simulink model "eg_6_05_R2020a"  (R2020a)
settings: Solver=ode4  StartTime=0.0  StopTime=1  FixedStep=0.001  RelTol=1e-3  EnableMultiTasking=on
values from neighbouring files (symbols this model uses):
  A = [ 0  1  0  0 ... (first row only)    [eg_6_02.m]    (also in eg_6_03.m = [ 0   1; eg_6_04_1a.m = [ 0   1; eg_6_04_1b.m = [ 0   1; eg_6_04_1c.m = [ 0   1)
  Av = [    0       1       0       0 ... (first row only)    [eg_6_05c.m]    (also in eg_6_05d.m)
  B = [  0 ... (first row only)    [eg_6_05a.m]    (also in eg_6_05b.m; eg_6_05c.m; eg_6_05d.m)
  Bv = [  0 ... (first row only)    [eg_6_05c.m]    (also in eg_6_05d.m)
  C = [ 0  0  1  0 ]    [eg_6_05a.m]    (also in eg_6_05b.m; eg_6_05c.m; eg_6_05d.m)
  H = 10    [eg_6_05c.m]    (also in eg_6_05d.m)
  K = [ -7/2  -5/2  -13/2  -11/2 ]    [eg_6_05c.m]    (also in eg_6_05d.m)
  L = - Delta_A*inv(Vo)*e'    [eg_6_05a.m]    (also in eg_6_05b.m = Kd'; eg_6_05c.m = Kd'; eg_6_05d.m = Kd')
  x0 = [ 1 ... (first row only)    [eg_6_04_1c.m]    (also in eg_6_05c.m = [ -0.5; eg_6_05d.m = [ -0.5)
  x0_hat = [ 0 ... (first row only)    [eg_6_04_1c.m]    (also in eg_6_05c.m; eg_6_05d.m)
settings Model: Creator=kawata  LastModifiedBy=kawata
settings DataIOCC: LimitDataPoints=on  SaveFormat=Array  SignalLoggingSaveFormat=ModelDataLogs  ReturnWorkspaceOutputs=off
settings OptimizationCC: ExpressionDepthLimit=2147483647  LifeSpan=inf
settings DebuggingCC: UnderspecifiedInitializationDetection=Classic  MergeDetectMultiDrivingBlocksExec=none  SolverPrmCheckMsg=warning  FcnCallInpInsideContextMsg=warning  StateNameClashWarn=warning  SFUnexpectedBacktrackingDiag=warning  SFNoUnconditionalDefaultTransitionDiag=warning  SFExecutionAtInitializationDiag=none  ArithmeticOperatorsInVariantConditions=warning
settings HardwareCC: ProdBitPerPointer=32  ProdBitPerSizeT=32  ProdBitPerPtrDiffT=32  ProdLargestAtomicFloat=None  ProdIntDivRoundTo=Undefined  ProdEndianess=Unspecified  ProdWordSize=32  ProdHWDeviceType=32-bit Generic
settings ModelReferenceCC: PropagateSignalLabelsOutOfModel=off
settings SFSimCC: SimUseLocalCustomCode=off  CustomCodeUndefinedFunction=UseInterfaceOnly
settings RTWCC: RTWUseLocalCustomCode=off
settings CodeAppCC: StateflowObjectComments=on
settings GRTTargetCC: TargetLangStandard=C89/C90 (ANSI)  CombineOutputUpdateFcns=off  GRTInterface=on
settings ConfigComp: CovMetricSettings=dw  CovSaveCumulativeToWorkspaceVar=on  CovSaveSingleToWorkspaceVar=on  CovExternalEMLEnable=off

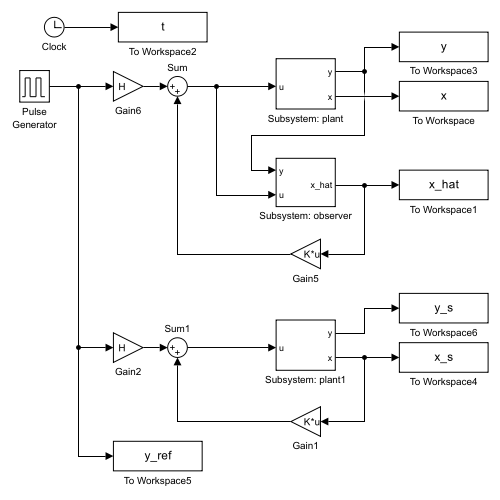
[thumbnail: Simulink's stored preview of the top-level diagram]
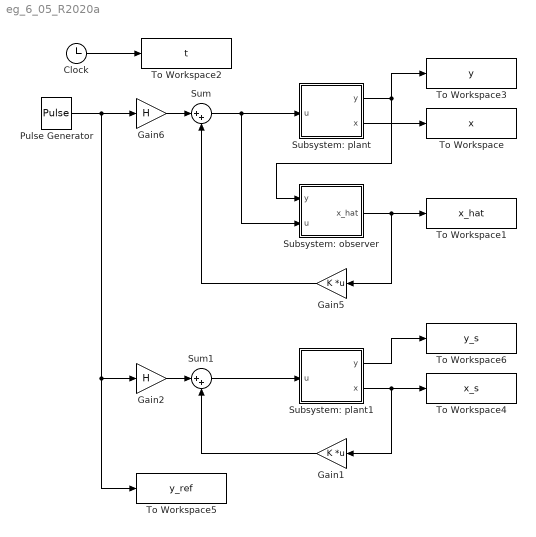
== system eg_6_05_R2020a ==
  Clock : Clock
  Gain1 : Gain  Gain=K  Multiplication=Matrix(K*u)
  Gain2 : Gain  Gain=H
  Gain5 : Gain  Gain=K  Multiplication=Matrix(K*u)
  Gain6 : Gain  Gain=H
  Pulse Generator : DiscretePulseGenerator  PulseType=Time based  Period=10  PulseWidth=50
  Subsystem: observer : Subsystem
  Subsystem: plant : Subsystem
  Subsystem: plant1 : Subsystem
  Sum : Sum  Inputs=|++  InputSameDT=on  SaturateOnIntegerOverflow=on  OutDataTypeStr=Inherit: Same as first input
  Sum1 : Sum  Inputs=|++  InputSameDT=on  SaturateOnIntegerOverflow=on  OutDataTypeStr=Inherit: Same as first input
  To Workspace : ToWorkspace  VariableName=x  SampleTime=-1
  To Workspace1 : ToWorkspace  VariableName=x_hat  SampleTime=-1
  To Workspace2 : ToWorkspace  VariableName=t  SampleTime=-1
  To Workspace3 : ToWorkspace  VariableName=y  SampleTime=-1
  To Workspace4 : ToWorkspace  VariableName=x_s  SampleTime=-1
  To Workspace5 : ToWorkspace  VariableName=y_ref  SampleTime=-1
  To Workspace6 : ToWorkspace  VariableName=y_s  SampleTime=-1
  wires:
  Clock/1 -> To Workspace2/1
  Sum/1 -> Subsystem: observer/2(u), Subsystem: plant/1(u)
  Subsystem: observer/1(x_hat) -> To Workspace1/1, Gain5/1
  Subsystem: plant/2(x) -> To Workspace/1
  Subsystem: plant/1(y) -> To Workspace3/1, Subsystem: observer/1(y)
  Pulse Generator/1 -> Gain6/1, To Workspace5/1, Gain2/1
  Gain6/1 -> Sum/1
  Gain5/1 -> Sum/2
  Sum1/1 -> Subsystem: plant1/1(u)
  Subsystem: plant1/2(x) -> To Workspace4/1, Gain1/1
  Subsystem: plant1/1(y) -> To Workspace6/1
  Gain2/1 -> Sum1/1
  Gain1/1 -> Sum1/2

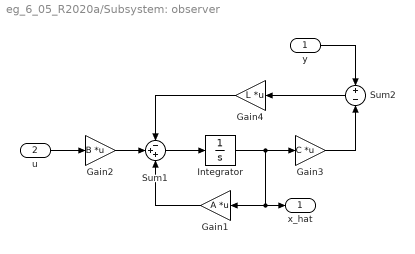
== system eg_6_05_R2020a/Subsystem: observer ==
  y : Inport
  u : Inport  Port=2
  Gain1 : Gain  Gain=A  Multiplication=Matrix(K*u)  SaturateOnIntegerOverflow=on  OutDataTypeStr=Inherit: Same as input  ParamDataTypeStr=Inherit: Same as input
  Gain2 : Gain  Gain=B  Multiplication=Matrix(K*u)  SaturateOnIntegerOverflow=on  OutDataTypeStr=Inherit: Same as input  ParamDataTypeStr=Inherit: Same as input
  Gain3 : Gain  Gain=C  Multiplication=Matrix(K*u)  SaturateOnIntegerOverflow=on  OutDataTypeStr=Inherit: Same as input  ParamDataTypeStr=Inherit: Same as input
  Gain4 : Gain  Gain=L  Multiplication=Matrix(K*u)  SaturateOnIntegerOverflow=on  OutDataTypeStr=Inherit: Same as input  ParamDataTypeStr=Inherit: Same as input
  Integrator : Integrator  InitialCondition=x0_hat
  Sum1 : Sum  Inputs=-++  InputSameDT=on  SaturateOnIntegerOverflow=on  OutDataTypeStr=Inherit: Same as first input
  Sum2 : Sum  Inputs=+|-  InputSameDT=on  SaturateOnIntegerOverflow=on  OutDataTypeStr=Inherit: Same as first input
  x_hat : Outport  VectorParamsAs1DForOutWhenUnconnected=off
  wires:
  u/1 -> Gain2/1
  y/1 -> Sum2/1
  Gain4/1 -> Sum1/1
  Sum2/1 -> Gain4/1
  Gain1/1 -> Sum1/3
  Gain2/1 -> Sum1/2
  Sum1/1 -> Integrator/1
  Integrator/1 -> Gain1/1, x_hat/1, Gain3/1
  Gain3/1 -> Sum2/2

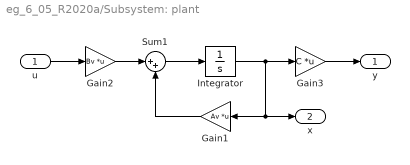
== system eg_6_05_R2020a/Subsystem: plant ==
  u : Inport
  Gain1 : Gain  Gain=Av  Multiplication=Matrix(K*u)  SaturateOnIntegerOverflow=on  OutDataTypeStr=Inherit: Same as input  ParamDataTypeStr=Inherit: Same as input
  Gain2 : Gain  Gain=Bv  Multiplication=Matrix(K*u)  SaturateOnIntegerOverflow=on  OutDataTypeStr=Inherit: Same as input  ParamDataTypeStr=Inherit: Same as input
  Gain3 : Gain  Gain=C  Multiplication=Matrix(K*u)  SaturateOnIntegerOverflow=on  OutDataTypeStr=Inherit: Same as input  ParamDataTypeStr=Inherit: Same as input
  Integrator : Integrator  InitialCondition=x0
  Sum1 : Sum  Inputs=|++  InputSameDT=on  SaturateOnIntegerOverflow=on  OutDataTypeStr=Inherit: Same as first input
  y : Outport  VectorParamsAs1DForOutWhenUnconnected=off
  x : Outport  Port=2  VectorParamsAs1DForOutWhenUnconnected=off
  wires:
  Integrator/1 -> Gain3/1, x/1, Gain1/1
  Sum1/1 -> Integrator/1
  u/1 -> Gain2/1
  Gain2/1 -> Sum1/1
  Gain1/1 -> Sum1/2
  Gain3/1 -> y/1

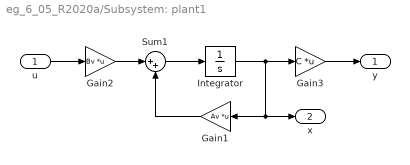
== system eg_6_05_R2020a/Subsystem: plant1 ==
  u : Inport
  Gain1 : Gain  Gain=Av  Multiplication=Matrix(K*u)  SaturateOnIntegerOverflow=on  OutDataTypeStr=Inherit: Same as input  ParamDataTypeStr=Inherit: Same as input
  Gain2 : Gain  Gain=Bv  Multiplication=Matrix(K*u)  SaturateOnIntegerOverflow=on  OutDataTypeStr=Inherit: Same as input  ParamDataTypeStr=Inherit: Same as input
  Gain3 : Gain  Gain=C  Multiplication=Matrix(K*u)  SaturateOnIntegerOverflow=on  OutDataTypeStr=Inherit: Same as input  ParamDataTypeStr=Inherit: Same as input
  Integrator : Integrator  InitialCondition=x0
  Sum1 : Sum  Inputs=|++  InputSameDT=on  SaturateOnIntegerOverflow=on  OutDataTypeStr=Inherit: Same as first input
  y : Outport  VectorParamsAs1DForOutWhenUnconnected=off
  x : Outport  Port=2  VectorParamsAs1DForOutWhenUnconnected=off
  wires:
  Integrator/1 -> Gain3/1, x/1, Gain1/1
  Sum1/1 -> Integrator/1
  u/1 -> Gain2/1
  Gain2/1 -> Sum1/1
  Gain1/1 -> Sum1/2
  Gain3/1 -> y/1
